simulink model "BE_EGAL_01"  (R2024b)
settings: Solver=ode45  StartTime=0.0  StopTime=Tfinal  RelTol=1e-3  EnableMultiTasking=on
undefined symbols (not defined in the file or in its folder): dfilt, Tfinal
libraries: commdigbbndam3 x2, commchan3 x1, dspobslib x1, commsink2 x1, commrandsrc3 x1
settings Model: Creator=Epsilon_2  LastModifiedBy=paulj
settings SolverCC: AlgebraicLoopSolver=TrustRegion
settings DataIOCC: LimitDataPoints=on  SaveFormat=Array  SignalLoggingSaveFormat=ModelDataLogs  SaveOutput=off  SaveTime=off  ReturnWorkspaceOutputs=off  SignalLoggingName=sigsOut
settings OptimizationCC: ExpressionDepthLimit=2147483647  InitFltsAndDblsToZero=on  LifeSpan=inf
settings DebuggingCC: SaveWithParameterizedLinksMsg=none  UnderspecifiedInitializationDetection=Classic  MergeDetectMultiDrivingBlocksExec=none  SignalResolutionControl=TryResolveAllWithWarning  MultiTaskDSMMsg=warning  MultiTaskCondExecSysMsg=none  FcnCallInpInsideContextMsg=warning  UnconnectedInputMsg=warning  UnconnectedOutputMsg=warning  UnconnectedLineMsg=warning  StateNameClashWarn=warning  SFUnexpectedBacktrackingDiag=warning  SFNoUnconditionalDefaultTransitionDiag=warning  SFExecutionAtInitializationDiag=none  ArithmeticOperatorsInVariantConditions=warning
settings HardwareCC: ProdBitPerPointer=32  ProdBitPerSizeT=32  ProdBitPerPtrDiffT=32  ProdLargestAtomicFloat=None  ProdIntDivRoundTo=Undefined  ProdEndianess=Unspecified  ProdWordSize=32  ProdHWDeviceType=32-bit Generic  TargetUnknown=on
settings ModelReferenceCC: PropagateSignalLabelsOutOfModel=off
settings RTWCC: GPUComputeCapability=3.5
settings CodeAppCC: StateflowObjectComments=on
settings GRTTargetCC: TargetFcnLib=ansi_tfl_tmw.mat  TargetLangStandard=C89/C90 (ANSI)  ModelReferenceCompliant=off  CombineOutputUpdateFcns=off  MatFileLogging=off  GRTInterface=on
settings ConfigComp: CovMetricSettings=dw  CovSaveCumulativeToWorkspaceVar=on  CovSaveSingleToWorkspaceVar=on

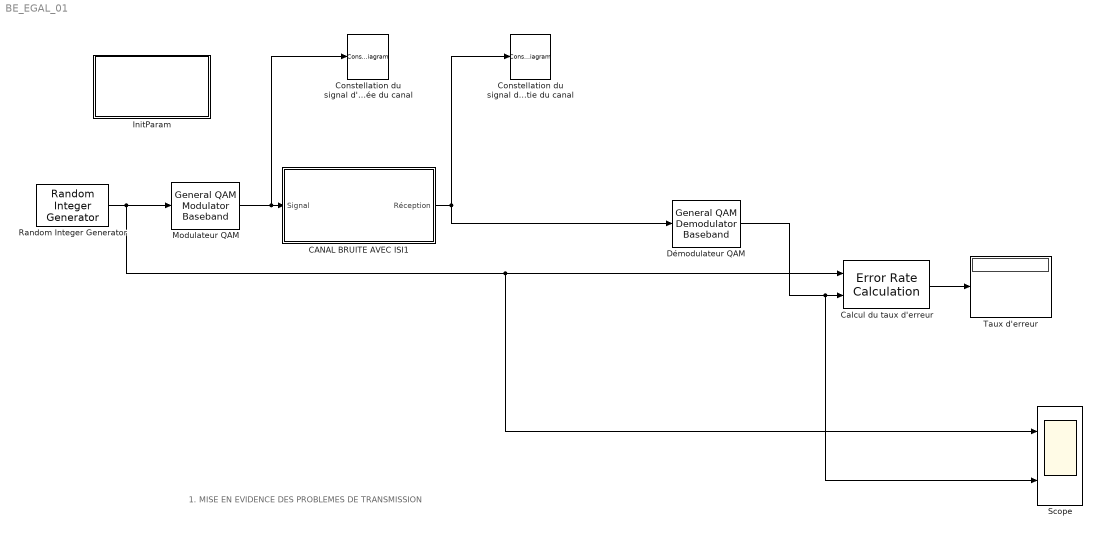
== system BE_EGAL_01 ==
  note: 1. MISE EN EVIDENCE DES PROBLEMES DE TRANSMISSION
  CANAL BRUITE AVEC ISI1 : Subsystem
  Calcul du taux d'erreur : commsink2/Error Rate Calculation  N=0  st_delay=0  cp_mode=Entire frame  subframe=[]  PMode=Port  WsName=ErrorVec  RsMode2=off  stop=off  numErr=100  maxBits=1e6
  Constellation du signal d'entrée du canal : ConstellationDiagram  Tag=ScatterPlot  WindowPosition=[333.000000,149.000000,600.000000,600.000000,]  Visible=on  ScopeFrameLocation=window  SymbolsToDisplaySource=Property  SymbolsToDisplay=Tfinal  XLimits=[-1.47,1.47]  YLimits=[-1.38,1.38]  FigPos=[232 118 560 560]
  Constellation du signal de sortie du canal : ConstellationDiagram  Tag=ScatterPlot  WindowPosition=[1069.000000,138.000000,600.000000,600.000000,]  Visible=on  ScopeFrameLocation=window  SymbolsToDisplaySource=Property  SymbolsToDisplay=Tfinal  XLimits=[-1.47,1.47]  YLimits=[-1.38,1.38]  FigPos=[232 118 560 560]
  "Démodulateur QAM " : commdigbbndam3/General QAM Demodulator Baseband  SigCon=Constellation  OutType=Integer  DecType=Hard decision  VarSource=Dialog  Variance=1  outDtypeBit=Inherit via internal rule  outDtype=double  roundingMode=Floor  overflowMode=Wrap  OvFlMode=off  OvFlModeLastStrValue=off  sigConstWordLen=16  sigConstDataTypeStr=Inherit: Same word length as input  sigConstLastDataTypeStr=Inherit: Same word length as input  accum1WordLen=32  accum1FracLen=30  prodInWordLen=32  prodInFracLen=30  prodInDataTypeStr=Inherit: Same as accumulator 1  prodInLastDataTypeStr=Inherit: Same as accumulator 1  prodOutWordLen=32  prodOutFracLen=30  accum2WordLen=32  accum2FracLen=30  accum3WordLen=32  accum3FracLen=30  nsiWordLen=32  nsiFracLen=30  nsiDataTypeStr=Inherit: Same as accumulator 3  nsiLastDataTypeStr=Inherit: Same as accumulator 3  invn0WordLen=16  invn0FracLen=8  invn0DataTypeStr=Inherit: Same word length as input  invn0LastDataTypeStr=Inherit: Same word length as input  outputWordLen=32  outputFracLen=30
  InitParam : Subsystem  mask{Tech=1, Tfinal=Tfinal, Mconst=4, NumCanal=1, SNRcanal=20, NCoeffs=9, Kegal=0.02}
      mask prompts: Tech "Période de symbole"; Tfinal "Temps de simulation"; Mconst "Taille de la constellation de la modulation QAM : M (2^k)"; NumCanal "Modele RIF du canal"; SNRcanal "SNR du canal (en dB)"; NCoeffs "Nb de coefficients de l'égalisateur"; Kegal "Gain de l'égalisateur"
      mask help: Use the following mask to select the different parameters for the simulation.
      mask init:
      | eStr = init_ISI(gcb);
      mask Display: disp('Initialisation')
  "Modulateur QAM " : commdigbbndam3/General QAM Modulator Baseband  SigCon=Constellation  outDtype=double  outWordLen=16  outUDDataType=sfix(16)  outFracLenMode=Best precision  outFracLen=15  outDataTypeStr=double  outLastDataTypeStr=double
  Random Integer Generator : commrandsrc3/Random Integer Generator  SetSize=4  SeedSource=Auto  Seed=0  SampleTime=1  SamplesPerFrame=1  OutputDataType=double  SimulateUsing=Interpreted execution
  Scope : Scope  NumInputPorts=2
  Taux d'erreur : Display
  wires:
  Random Integer Generator/1 -> "Modulateur QAM "/1, Calcul du taux d'erreur/1, Scope/1
  "Modulateur QAM "/1 -> Constellation du signal d'entrée du canal/1, CANAL BRUITE AVEC ISI1/1(Signal)
  Calcul du taux d'erreur/1 -> Taux d'erreur/1
  "Démodulateur QAM "/1 -> Calcul du taux d'erreur/2, Scope/2
  CANAL BRUITE AVEC ISI1/1(Réception) -> Constellation du signal de sortie du canal/1, "Démodulateur QAM "/1

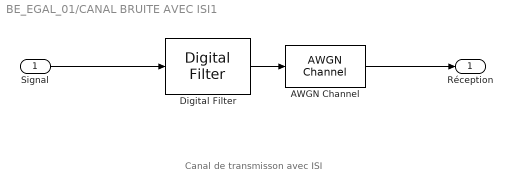
== system BE_EGAL_01/CANAL BRUITE AVEC ISI1 ==
  note: Canal de transmisson avec ISI
  Signal : Inport
  AWGN Channel : commchan3/AWGN Channel  LegacyMode=on  NoiseMethod="Signal to noise ratio  (SNR)"  noiseMode="Signal to noise ratio  (SNR)"  EbNo=10  EsNo=10  SNR=SNRcanal  BitsPerSymbol=1  SignalPower=1  SamplesPerSymbol=1  SymbolPeriod=1  VarianceSource=Parameter  Variance=1  RandomStream=Global stream  Seed=67  SimulateUsing=Code generation
  Digital Filter : dspobslib/Digital Filter  TypePopup=FIR (all zeros)  IIRFiltStruct=Direct form II transposed  AllPoleFiltStruct=Direct form  FIRFiltStruct=Direct form  CoeffSource=Specify via dialog  NumCoeffs=NumCanal  DenCoeffs=[1 0.1]  BiQuadCoeffs=[1 0.3 0.4 1 0.1 0.2]  LatticeCoeffs=[0.2 0.4]  denIgnore=on  FiltPerSampPopup=One filter per sample  IC=0  ICnum=0  ICden=0  roundingMode=Floor  overflowMode=off  ScaleValues=1  scaleValueFracLength=14  stageInFracLength=15  stageOutFracLength=15  FilterSource=Specify via dialog  dfiltObjectName=dfilt.dffir([1 2 1])  InputProcessing=Columns as channels (frame based)
  Réception : Outport
  wires:
  Signal/1 -> Digital Filter/1
  AWGN Channel/1 -> Réception/1
  Digital Filter/1 -> AWGN Channel/1

== system BE_EGAL_01/InitParam ==
